simulink library "csu_valvesim_signal_interface_lib"  (R2014b)
settings: Solver=ode45  StartTime=0.0  StopTime=10.0  RelTol=1e-3
settings Model: Creator=escrane  LastModifiedBy=mstewart

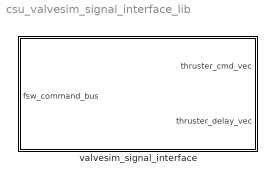
== system csu_valvesim_signal_interface_lib ==
  valvesim_signal_interface : Subsystem

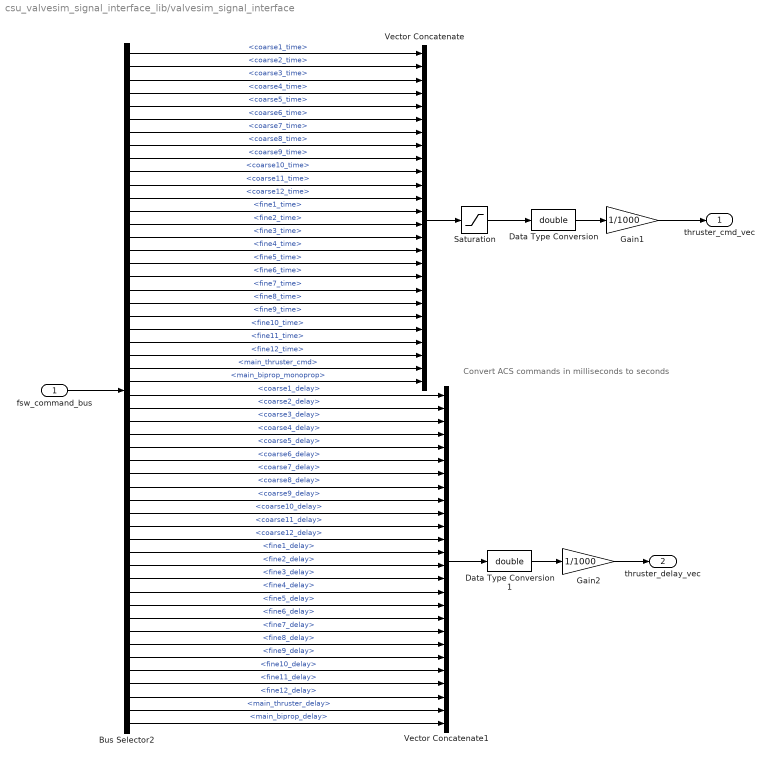
== system csu_valvesim_signal_interface_lib/valvesim_signal_interface ==
  note: Convert ACS commands in milliseconds to seconds
  fsw_command_bus : Inport
  Bus Selector2 : BusSelector  OutputSignals=act_bus_msg.coarse1_time,act_bus_msg.coarse2_time,act_bus_msg.coarse3_time,act_bus_msg.coarse4_time,act_bus_msg.coarse5_time,act_bus_msg.coarse6_time,act_bus_msg.coarse7_time,act_bus_msg.coarse8_time,act_bus_msg.coarse9_time,act_bus_msg.coarse10_time,act_bus_msg.coarse11_time,act_bus_msg.coarse12_time,act_bus_msg.fine1_time,act_bus_msg.fine2_time,act_bus_msg.fine3_time,act_bus_msg.fine4_time,act_bus_msg.fine5_time,act_bus_msg.fine6_time,act_bus_msg.fine7_time,act_bus_msg.fine8_time,act_bus_msg.fine9_time,act_bus_msg.fine10_time,act_bus_msg.fine11_time,act_bus_msg.fine12_time,act_bus_msg.main_thruster_cmd,act_bus_msg.main_biprop_monoprop,act_bus_msg.coarse1_delay,act_bus_msg.coarse2_delay,act_bus_msg.coarse3_delay,act_bus_msg.coarse4_delay,act_bus_msg.coarse5_delay,act_bus_msg.coarse6_delay,act_bus_msg.coarse7_delay,act_bus_msg.coarse8_delay,act_bus_msg.coarse9_delay,act_bus_msg.coarse10_delay,act_bus_msg.coarse11_delay,act_bus_msg.coarse12_delay,act_bus_msg.fine1_delay,act_bus_msg.fine2_delay,act_bus_msg.fine3_delay,act_bus_msg.fine4_delay,act_bus_msg.fine5_delay,act_bus_msg.fine6_delay,act_bus_msg.fine7_delay,act_bus_msg.fine8_delay,act_bus_msg.fine9_delay,act_bus_msg.fine10_delay,act_bus_msg.fine11_delay,act_bus_msg.fine12_delay,act_bus_msg.main_thruster_delay,act_bus_msg.main_biprop_delay
  Data Type Conversion : DataTypeConversion  OutDataTypeStr=double
  Data Type Conversion1 : DataTypeConversion  OutDataTypeStr=double
  Gain1 : Gain  Gain=1/1000  OutDataTypeStr=double
  Gain2 : Gain  Gain=1/1000  OutDataTypeStr=double
  Saturation : Saturate  UpperLimit=100  LowerLimit=0
  Vector Concatenate : Concatenate  NumInputs=26
  Vector Concatenate1 : Concatenate  NumInputs=26
  thruster_cmd_vec : Outport
  thruster_delay_vec : Outport  Port=2
  wires:
  Vector Concatenate1/1 -> Data Type Conversion1/1
  Gain2/1 -> thruster_delay_vec/1
  Data Type Conversion1/1 -> Gain2/1
  Bus Selector2/50 -> Vector Concatenate1/24  "<fine12_delay>"
  Bus Selector2/44 -> Vector Concatenate1/18  "<fine6_delay>"
  Bus Selector2/51 -> Vector Concatenate1/25  "<main_thruster_delay>"
  Bus Selector2/15 -> Vector Concatenate/15  "<fine3_time>"
  Bus Selector2/14 -> Vector Concatenate/14  "<fine2_time>"
  Bus Selector2/12 -> Vector Concatenate/12  "<coarse12_time>"
  Bus Selector2/11 -> Vector Concatenate/11  "<coarse11_time>"
  Bus Selector2/16 -> Vector Concatenate/16  "<fine4_time>"
  Bus Selector2/9 -> Vector Concatenate/9  "<coarse9_time>"
  Bus Selector2/8 -> Vector Concatenate/8  "<coarse8_time>"
  Bus Selector2/7 -> Vector Concatenate/7  "<coarse7_time>"
  Bus Selector2/6 -> Vector Concatenate/6  "<coarse6_time>"
  Bus Selector2/13 -> Vector Concatenate/13  "<fine1_time>"
  Bus Selector2/4 -> Vector Concatenate/4  "<coarse4_time>"
  Bus Selector2/10 -> Vector Concatenate/10  "<coarse10_time>"
  Bus Selector2/3 -> Vector Concatenate/3  "<coarse3_time>"
  Bus Selector2/2 -> Vector Concatenate/2  "<coarse2_time>"
  Bus Selector2/5 -> Vector Concatenate/5  "<coarse5_time>"
  Bus Selector2/1 -> Vector Concatenate/1  "<coarse1_time>"
  Bus Selector2/21 -> Vector Concatenate/21  "<fine9_time>"
  Bus Selector2/20 -> Vector Concatenate/20  "<fine8_time>"
  Bus Selector2/19 -> Vector Concatenate/19  "<fine7_time>"
  Bus Selector2/18 -> Vector Concatenate/18  "<fine6_time>"
  Bus Selector2/17 -> Vector Concatenate/17  "<fine5_time>"
  Bus Selector2/26 -> Vector Concatenate/26  "<main_biprop_monoprop>"
  Bus Selector2/25 -> Vector Concatenate/25  "<main_thruster_cmd>"
  Bus Selector2/24 -> Vector Concatenate/24  "<fine12_time>"
  Bus Selector2/23 -> Vector Concatenate/23  "<fine11_time>"
  Bus Selector2/22 -> Vector Concatenate/22  "<fine10_time>"
  Bus Selector2/41 -> Vector Concatenate1/15  "<fine3_delay>"
  Bus Selector2/31 -> Vector Concatenate1/5  "<coarse5_delay>"
  Bus Selector2/33 -> Vector Concatenate1/7  "<coarse7_delay>"
  Bus Selector2/49 -> Vector Concatenate1/23  "<fine11_delay>"
  Bus Selector2/52 -> Vector Concatenate1/26  "<main_biprop_delay>"
  Bus Selector2/36 -> Vector Concatenate1/10  "<coarse10_delay>"
  Bus Selector2/29 -> Vector Concatenate1/3  "<coarse3_delay>"
  Bus Selector2/39 -> Vector Concatenate1/13  "<fine1_delay>"
  Bus Selector2/37 -> Vector Concatenate1/11  "<coarse11_delay>"
  Bus Selector2/48 -> Vector Concatenate1/22  "<fine10_delay>"
  Bus Selector2/38 -> Vector Concatenate1/12  "<coarse12_delay>"
  Bus Selector2/32 -> Vector Concatenate1/6  "<coarse6_delay>"
  Bus Selector2/27 -> Vector Concatenate1/1  "<coarse1_delay>"
  Bus Selector2/30 -> Vector Concatenate1/4  "<coarse4_delay>"
  Bus Selector2/35 -> Vector Concatenate1/9  "<coarse9_delay>"
  Bus Selector2/34 -> Vector Concatenate1/8  "<coarse8_delay>"
  Bus Selector2/28 -> Vector Concatenate1/2  "<coarse2_delay>"
  Bus Selector2/46 -> Vector Concatenate1/20  "<fine8_delay>"
  Bus Selector2/43 -> Vector Concatenate1/17  "<fine5_delay>"
  Bus Selector2/40 -> Vector Concatenate1/14  "<fine2_delay>"
  Bus Selector2/45 -> Vector Concatenate1/19  "<fine7_delay>"
  Bus Selector2/42 -> Vector Concatenate1/16  "<fine4_delay>"
  Bus Selector2/47 -> Vector Concatenate1/21  "<fine9_delay>"
  Gain1/1 -> thruster_cmd_vec/1
  Vector Concatenate/1 -> Saturation/1
  fsw_command_bus/1 -> Bus Selector2/1
  Data Type Conversion/1 -> Gain1/1
  Saturation/1 -> Data Type Conversion/1
